simulink model "Motor_pos0"  (R2020b)
settings: Solver=ode15s  StartTime=0.0  StopTime=0.2  RelTol=1e-3
values from neighbouring files (symbols this model uses):
  b = 3.5077E-6    [motor_pos.sldd]
  J = 3.2284E-6    [motor_pos.sldd]
  K = 0.0274    [motor_pos.sldd]
  L = 2.75E-6    [motor_pos.sldd]
  R = 4.0    [motor_pos.sldd]
settings Model: DataDictionary=motor_pos.sldd  Creator=priyaD  LastModifiedBy=priyaD
settings DataIOCC: SaveOutput=off  SaveTime=off

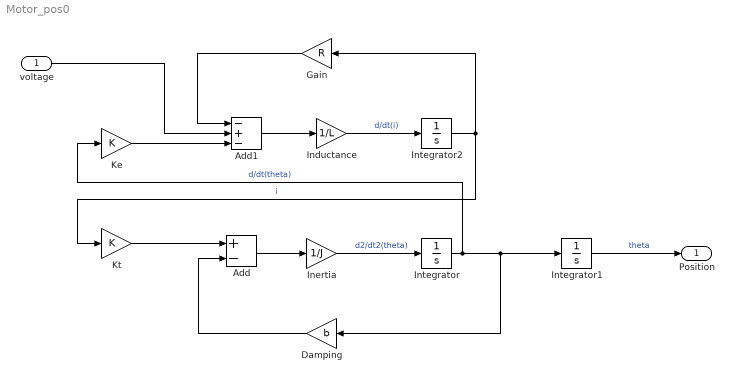
== system Motor_pos0 ==
  voltage : Inport  OutDataTypeStr=double  PortDimensions=1  SampleTime=0
  Add : Sum  Inputs=+-
  Add1 : Sum  Inputs=-+-
  Damping : Gain  Gain=b
  Gain : Gain  Gain=R
  Inductance : Gain  Gain=1/L
  Inertia : Gain  Gain=1/J
  Integrator : Integrator
  Integrator1 : Integrator
  Integrator2 : Integrator
  Ke : Gain  Gain=K
  Kt : Gain  Gain=K
  Position : Outport  OutDataTypeStr=double  PortDimensions=1  SampleTime=0
  wires:
  Damping/1 -> Add/2
  Integrator/1 -> Integrator1/1, Damping/1, Ke/1  "d/dt(theta)"
  Gain/1 -> Add1/1
  Add/1 -> Inertia/1
  Kt/1 -> Add/1
  Inertia/1 -> Integrator/1  "d2/dt2(theta)"
  Add1/1 -> Inductance/1
  voltage/1 -> Add1/2
  Integrator2/1 -> Kt/1, Gain/1  "i"
  Ke/1 -> Add1/3
  Inductance/1 -> Integrator2/1  "d/dt(i)"
  Integrator1/1 -> Position/1  "theta"
